simulink model "environment"  (Simulink 8.1)
settings: Solver=ode45  StartTime=0.0  StopTime=10.0  RelTol=1e-3
settings Model: Creator=eiseles  LastModifiedBy=eiseles
settings DataIOCC: SignalLoggingSaveFormat=Dataset
settings OptimizationCC: ExpressionDepthLimit=128
settings DebuggingCC: FcnCallInpInsideContextMsg=EnableAllAsError
settings GRTTargetCC: CombineOutputUpdateFcns=on  GRTInterface=off

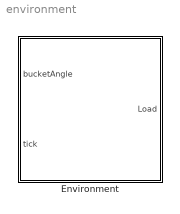
== system environment ==
  Environment : Subsystem

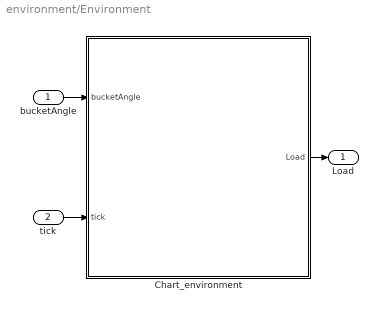
== system environment/Environment ==
  bucketAngle : Inport
  tick : Inport  Port=2
  Chart_environment : Stateflow chart  TreatAsAtomicUnit=on
  Load : Outport
  wires:
  bucketAngle/1 -> Chart_environment/1(bucketAngle)
  Chart_environment/1(Load) -> Load/1
  tick/1 -> Chart_environment/2(tick)

== stateflow chart Environment/Chart_environment ==
  state loaded
    en:
    Load = 2000;
  state unloading
    en:
    Load = 2000;
    du:
    Load = Load - .1*Load;
  state unloaded
    en:
    Load = 0;
  loaded -> unloading : [-bucketAngle<=.6]
  (default) -> loaded
  unloading -> unloaded : [Load <= 10 ]
  data: bucketAngle input double; Load output double; tick input double
